simulink model "sistemas_tarea2"  (R2018a)
settings: Solver=VariableStepAuto  StartTime=0.0  StopTime=400  RelTol=1e-3
settings Model: Creator=carma  LastModifiedBy=carma

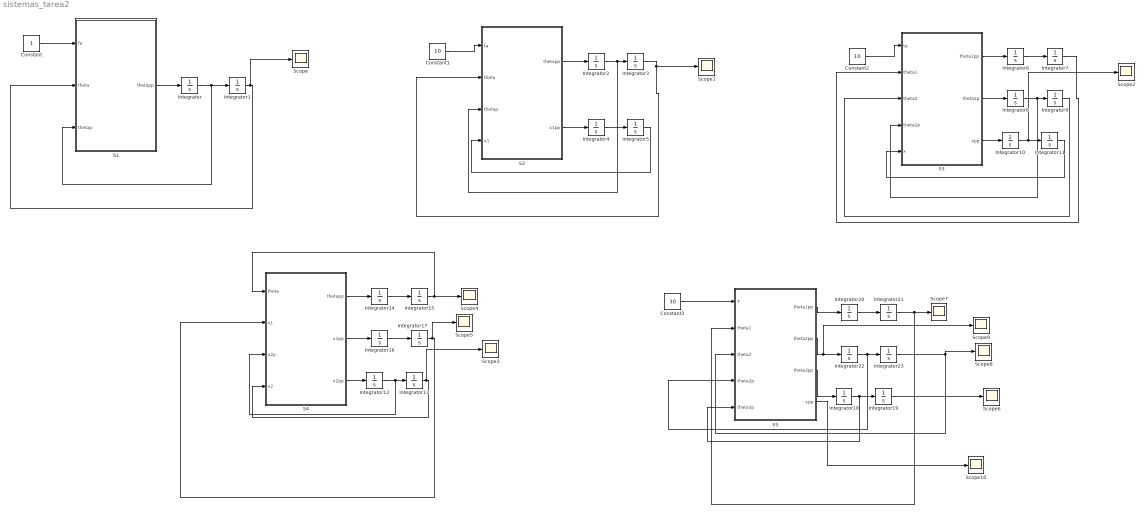
== system sistemas_tarea2 ==
  Constant : Constant
  Constant1 : Constant  Value=10
  Constant2 : Constant  Value=10
  Constant3 : Constant  Value=30
  Integrator{,1..23} (24 alike) : Integrator
  S1 : MATLAB Function  TreatAsAtomicUnit=on
  S2 : MATLAB Function  TreatAsAtomicUnit=on
  S3 : MATLAB Function  TreatAsAtomicUnit=on
  S4 : MATLAB Function  TreatAsAtomicUnit=on
  S5 : MATLAB Function  TreatAsAtomicUnit=on
  Scope{,1..10} (11 alike) : Scope
  wires:
  S1/1(thetapp) -> Integrator/1
  Integrator/1 -> S1/3(thetap), Integrator1/1
  Integrator1/1 -> Scope/1, S1/2(theta)
  Constant/1 -> S1/1(fa)
  S2/1(thetapp) -> Integrator2/1
  Integrator3/1 -> S2/2(theta), Scope1/1
  Constant1/1 -> S2/1(fa)
  Integrator2/1 -> S2/3(thetap), Integrator3/1
  S2/2(x1pp) -> Integrator4/1
  Integrator4/1 -> Integrator5/1
  Integrator5/1 -> S2/4(x1)
  S3/1(theta1pp) -> Integrator6/1
  Integrator6/1 -> Integrator7/1
  Constant2/1 -> S3/1(ta)
  Integrator8/1 -> S3/4("theta2p "), Integrator9/1
  Integrator7/1 -> S3/2(theta1)
  S3/2(theta2p) -> Integrator8/1
  Integrator9/1 -> S3/3(theta2)
  Integrator10/1 -> Scope2/1, Integrator11/1
  S3/3(xpp) -> Integrator10/1
  Integrator11/1 -> S3/5(x)
  Integrator12/1 -> S4/3(x2p), Integrator13/1
  S4/3(x2pp) -> Integrator12/1
  Integrator16/1 -> Integrator17/1
  Integrator14/1 -> Integrator15/1
  S4/2(x1pp) -> Integrator16/1
  S4/1(thetapp) -> Integrator14/1
  Integrator15/1 -> Scope4/1, S4/1(theta)
  Integrator17/1 -> Scope5/1, S4/2(x1)
  Integrator13/1 -> Scope3/1, S4/4(x2)
  Integrator21/1 -> S5/2(theta1), Scope7/1
  S5/1(theta1pp) -> Integrator20/1
  Integrator22/1 -> S5/4(theta2p), Integrator23/1
  S5/3(theta3pp) -> Integrator18/1
  Integrator20/1 -> Integrator21/1
  Integrator19/1 -> Scope6/1
  S5/2(theta2pp) -> Scope9/1, Integrator22/1
  Integrator18/1 -> S5/5(theta3p), Integrator19/1
  Constant3/1 -> S5/1(T)
  Integrator23/1 -> Scope8/1, S5/3(theta2)
  S5/4(xpp) -> Scope10/1

== matlab function sistemas_tarea2/S2 ==
  data: fa input; thetapp output; theta input; thetap input; x1 input; x1pp output
function [thetapp,x1pp] = fcn(fa,theta,thetap,x1)
%Parametros
M=10;
g=9.8;
J=70;
B=14;
R=0.1;
K1=200;
K2=130;

K1 = 469.34;
K2 = 200;
R = 0.1;
% R2 = R^2;
B = 50;
J = 0.15;
M = 50;
g = 9.8;
%Ecuaciones

% x2pp=fa+M*g-K1*x2-T;
x2=R*theta;
% x2pp=R*thetapp;
% T=fa+M*g-K1*x2-x2pp*M;
thetapp=(-B*thetap+(fa+M*g-K1*x2)*R-K2*R*(R*theta-x1))/(J+M*R^2);
x1pp=-K2*(x1-R*theta)-M*g;

== matlab function sistemas_tarea2/S1 ==
  data: fa input; thetapp output; theta input; thetap input
function thetapp = fcn(fa,theta,thetap)
%Parametros
M=10;
g=9.8;
J=0.2;
B=14;
R=0.1;
K=200;

K=5;
B=2;
J=5;
R=1;
M=4;

%Ecuaciones

thetapp=(-B*thetap+(fa+M*g)*R-K*R^2*theta)/(J+M*R^2);

== matlab function sistemas_tarea2/S3 ==
  data: ta input; theta1pp output; theta1 input; theta2 input; theta2p input; theta2p output; x input; xpp output
function [theta1pp,theta2p, xpp] = fcn(ta,theta1,theta2,theta2p,x)
%Parametros
M=10;
g=9.8;
J1=20;
J2=10;
B=14;
R=0.1;
K1=20;
K2=130;
%Ecuaciones
xpp=(-K2*(x-R*theta2)-M*g)/M;
theta1pp=(ta-K1*(theta1-theta2))/J1;
theta2pp=(-B*theta2p+K2*R*(x-R*theta2)+K1*(theta1-theta2))/J2;

== matlab function sistemas_tarea2/S4 ==
  data: theta input; thetapp output; x1 input; x1pp output; x2p input; x2pp output; x2 input
function [thetapp,x1pp, x2pp] = fcn(theta,x1,x2p,x2)
%Parametros
M1=200;
M2=1;
g=9.8;
J1=20;
B=4400;
R1=0.2;
R2=0.05;
K1=7000;
K2=230;
K3=300;

M1=50;
M2=200;
J1=40;
B1=4000;
K1=1000;
K2=7000;
K3=400;
R1=0.5;
R2=0.1;



%Ecuaciones
thetaA=x2/R2;
x1pp=(M1*g-K1*(x1-R1*theta))/M1;
thetapp=(R1*K1*(x1-R1*theta)-K2*(theta-thetaA))/J1;
x2pp=(M2*g-2*K3*x2-B*x2p+K2*(theta-thetaA)/R2)/M2;

== matlab function sistemas_tarea2/S5 ==
  data: T input; theta1pp output; theta1 input; theta2pp output; theta2 input; theta3pp output; theta2p input; theta3p input; xpp output
function [theta1pp,theta2pp,theta3pp,xpp] = fcn(T,theta1,theta2,theta2p,theta3p)
%Parametros
M=20;
g=0*9.8;
J1=200;
J2=17;
J3=100;
D3=40;
B=23;
r=0.002;
K1=70;
K2=23;

J1 = 200; %kg*m^2
J2 = 10; %kg*m^2
J3 = 100; %kg*m^2
M = 10; %kg
K1 = 7000; %N*m/rad 
K2 = 10; %N/m
D3 = 400; %N*m*s/rad
fv = 230; %N*s/m 
r = 0.2; %m




%Ecuaciones

theta1pp=(T-K1*(theta1-theta2))/J1;
theta2pp=(K1*(theta1-theta2)-D3*(theta2p-theta3p)-r*(B*r*theta2p+K2*r*theta2-M*g))/(J2+M*r^2);
theta3pp=D3*(theta2p-theta3p)/J3;
xpp=r*theta2pp;
